simulink model "cstr_close"  (R2020b)
settings: Solver=ode15s  StartTime=0.0  StopTime=1200  RelTol=1e-8  EnableMultiTasking=on
libraries: simulink x10, pid_lib x1
settings Model: Creator=Karl  LastModifiedBy=Fuzz4
settings DataIOCC: SaveFormat=Array  ReturnWorkspaceOutputs=off  OutputOption=SpecifiedOutputTimes  OutputTimes=[0:1200]
settings OptimizationCC: LifeSpan=inf
settings DebuggingCC: UnderspecifiedInitializationDetection=Classic  MergeDetectMultiDrivingBlocksExec=none  SFUnexpectedBacktrackingDiag=warning  SFNoUnconditionalDefaultTransitionDiag=warning  SFExecutionAtInitializationDiag=none  ArithmeticOperatorsInVariantConditions=warning
settings HardwareCC: ProdBitPerPointer=32  ProdBitPerSizeT=32  ProdBitPerPtrDiffT=32  ProdLargestAtomicFloat=None  ProdIntDivRoundTo=Undefined  ProdEndianess=Unspecified  ProdWordSize=32  ProdHWDeviceType=32-bit Generic
settings ModelReferenceCC: PropagateSignalLabelsOutOfModel=off
settings SFSimCC: SimUseLocalCustomCode=off  CustomCodeUndefinedFunction=UseInterfaceOnly
settings RTWCC: RTWUseLocalCustomCode=off
settings CodeAppCC: StateflowObjectComments=on
settings GRTTargetCC: TargetLangStandard=C89/C90 (ANSI)
settings ConfigComp: CovMetricSettings=dw  CovSaveCumulativeToWorkspaceVar=on  CovSaveSingleToWorkspaceVar=on  CovExternalEMLEnable=off

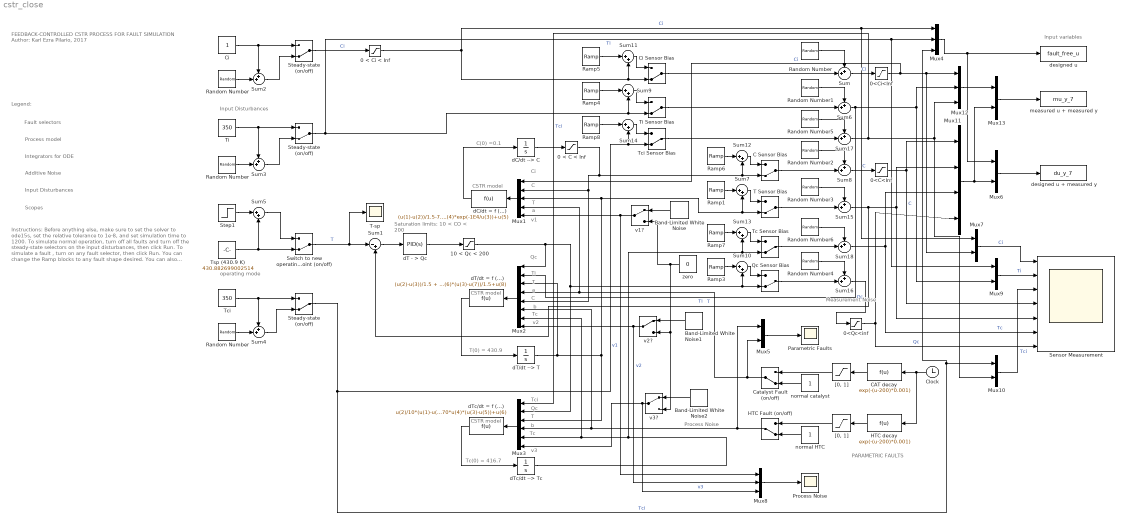
== system cstr_close ==
  note: Scopes
  note: Input Disturbances
  note: Instructions:
      |
      | Before anything else, make sure to set the solver to ode15s, set the relative tolerance to 1e-8, and set simulation time to 1200.
      |
      | To simulate normal operation, turn off all faults and turn off the steady-state selectors on the input disturbances, then click Run.
      |
      | To simulate a fault , turn on any fault selector, then click Run. You can change the Ramp blocks to any fault shape desired. You can also induce different disturbances by changing the Random Number blocks.
      |
      | Process Model:
  note: Additive Noise
  note: Integrators for ODE
  note: Process model
  note: Fault selectors
  note: Legend:
  note: FEEDBACK-CONTROLLED
      | CSTR PROCESS FOR
      | FAULT SIMULATION
      |
      | Author: Karl Ezra Pilario, 2017
  note: PARAMETRIC FAULTS
  note: v3
  note: v2
  note: v1
  note: Input variables
  note: T
  note: Tc(0) = 416.7
  note: Tc
  note: Qc
  note: Tc
  note: b
  note: Tci
  note: T
  note: Saturation limits:
      |  10 < CO < 200
  note: b
  note: CSTR model
  note: CSTR model
  note: T(0) = 430.9
  note: C(0) =0.1
  note: Measurement
      |         Noise
  note: Qc
  note: C
  note: a
  note: T
  note: Ti
  note: a
  note: C
  note: Ci
  note: CSTR model
  note: Process Noise
  note: Input Disturbances
  note: operating mode
  "   Steady-state (on/off)" : ManualSwitch  CurrentSetting=0
  "  Steady-state (on/off)" : ManualSwitch  CurrentSetting=0
  " Parametric Faults" : Scope
  " Process Noise" : Scope
  " Random Number" : RandomNumber  Seed=randi(100000)  SampleTime=60
  " [0, 1]" : Saturate  UpperLimit=1  LowerLimit=0
  0 < C < Inf : Saturate  UpperLimit=Inf  LowerLimit=0
  0 < Ci < Inf : Saturate  UpperLimit=Inf  LowerLimit=0
  0<C<Inf : Saturate  UpperLimit=Inf  LowerLimit=0
  0<Ci<Inf : Saturate  UpperLimit=Inf  LowerLimit=0
  0<Qc<inf : Saturate  UpperLimit=Inf  LowerLimit=0
  10 < Qc < 200 : Saturate  UpperLimit=200  LowerLimit=10
  Band-Limited White Noise : simulink/Sources/Band-Limited White Noise  Cov=[1e-4]  Ts=1  seed=randi(100000)
  Band-Limited White Noise1 : simulink/Sources/Band-Limited White Noise  Cov=[1e-4]  Ts=1  seed=randi(100000)
  Band-Limited White Noise2 : simulink/Sources/Band-Limited White Noise  Cov=[1e-4]  Ts=1  seed=randi(100000)
  C Sensor Bias : ManualSwitch  CurrentSetting=0
  CAT decay : Fcn  Expr=exp(-(u-200)*0.001)
  Catalyst Fault (on/off) : ManualSwitch  CurrentSetting=0
  Ci : Constant
  Ci Sensor Bias : ManualSwitch  CurrentSetting=0
  Clock : Clock
  HTC Fault (on/off) : ManualSwitch  CurrentSetting=0
  HTC decay : Fcn  Expr=exp(-(u-200)*0.001)
  Mux1 : Mux  Inputs=5
  Mux{5..7,9..10,13} (6 alike) : Mux  Inputs=2
  Mux11 : Mux
  Mux12 : Mux  Inputs=3
  Mux2 : Mux  Inputs=8
  Mux3 : Mux  Inputs=6
  Mux4 : Mux  Inputs=3
  Mux8 : Mux  Inputs=3
  Qc Sensor Bias : ManualSwitch  CurrentSetting=0
  Ramp1 : simulink/Sources/Ramp  slope=50/(1200-200)  start=200  InitialOutput=0
  Ramp3 : simulink/Sources/Ramp  slope=-100/(1200-200)  start=200  InitialOutput=0
  Ramp4 : simulink/Sources/Ramp  slope=150/(1200-200)  start=200  InitialOutput=0
  Ramp5 : simulink/Sources/Ramp  slope=2/(1200-200)  start=200  InitialOutput=0
  Ramp6 : simulink/Sources/Ramp  slope=1/(1200-200)  start=200  InitialOutput=0
  Ramp7 : simulink/Sources/Ramp  slope=50/(1200-200)  start=200  InitialOutput=0
  Ramp8 : simulink/Sources/Ramp  slope=100/(1200-200)  start=200  InitialOutput=0
  Random Number : RandomNumber  Variance=0.000001  Seed=randi(100000)  SampleTime=1
  Random Number1 : RandomNumber  Variance=0.05  Seed=randi(100000)  SampleTime=1
  Random Number2 : RandomNumber  Variance=0.000001  Seed=randi(100000)  SampleTime=1
  Random Number3 : RandomNumber  Variance=0.001  Seed=randi(100000)  SampleTime=1
  Random Number4 : RandomNumber  Variance=0.2  Seed=randi(100000)  SampleTime=1
  Random Number5 : RandomNumber  Variance=0.05  Seed=randi(100000)  SampleTime=1
  Random Number6 : RandomNumber  Variance=0.05  Seed=randi(100000)  SampleTime=1
  Random Number : RandomNumber  Variance=0.5  Seed=randi(100000)  SampleTime=60
  Random Number : RandomNumber  Variance=0.002  Seed=randi(100000)  SampleTime=60
  "Sensor Measurement " : Scope  NumInputPorts=7
  Steady-state (on/off) : ManualSwitch  CurrentSetting=0
  Step1 : Step  Time=300  After=10  SampleTime=0
  Sum{,2..4,6,8,15..18} (10 alike) : Sum  Inputs=++|
  Sum1 : Sum  Inputs=|-+
  Sum{5,7,9..14} (8 alike) : Sum  Inputs=|++
  Switch to new operating point (on/off) : ManualSwitch  CurrentSetting=0
  T Sensor Bias : ManualSwitch  CurrentSetting=0
  T-sp : Scope
  Tc Sensor Bias : ManualSwitch  CurrentSetting=0
  Tci : Constant  Value=350
  Tci Sensor Bias : ManualSwitch  CurrentSetting=0
  Ti : Constant  Value=350
  Ti Sensor Bias : ManualSwitch  CurrentSetting=0
  Tsp (430.9 K) : Constant  Value=430.882699002514
  "[0, 1]" : Saturate  UpperLimit=1  LowerLimit=0
  dC/dt --> C : Integrator  InitialCondition=0.1
  dC/dt = f (...) : Fcn  Expr=(u(1)-u(2))/1.5-7.2E10*u(2)*u(4)*exp(-1E4/u(3))+u(5)
  dT - > Qc : pid_lib/PID Controller  Controller=PID  Form=Parallel  TimeDomain=Continuous-time  UseExternalTs=off  SampleTime=-1  IntegratorMethod=Forward Euler  FilterMethod=Forward Euler  ControllerParametersSource=internal  P=1  I=5  D=0  UseFilter=on  N=100  TunerSelectOption=Transfer Function Based (PID Tuner App)  InitialConditionSource=internal  InitialConditionForIntegrator=148.550238092053  InitialConditionForFilter=0  DifferentiatorICPrevScaledInput=0  ExternalReset=none  TrackingMode=off  Kt=1  LimitOutput=on  SatLimitsSource=internal  UpperSaturationLimit=200  LowerSaturationLimit=10  LinearizeAsGain=on  AntiWindupMode=none  Kb=1  POutMin=[]  POutMax=[]  IOutMin=[]  IOutMax=[]  DOutMin=[]  DOutMax=[]  NOutMin=[]  NOutMax=[]  SumOutMin=[]  SumOutMax=[]  SaturationOutMin=[]  SaturationOutMax=[]  PParamMin=[]  PParamMax=[]  IParamMin=[]  IParamMax=[]  DParamMin=[]  DParamMax=[]  NParamMin=[]  NParamMax=[]  KbParamMin=[]  KbParamMax=[]  KtParamMin=[]  KtParamMax=[]  KbOutMin=[]  KbOutMax=[]  KtOutMin=[]  KtOutMax=[]  IntegratorOutMin=[]  IntegratorOutMax=[]  FilterOutMin=[]  FilterOutMax=[]  SumI1OutMin=[]  SumI1OutMax=[]  SumI2OutMin=[]  SumI2OutMax=[]  SumI3OutMin=[]  SumI3OutMax=[]  SumI4OutMin=[]  SumI4OutMax=[]  SumDOutMin=[]  SumDOutMax=[]  DifferentiatorOutMin=[]  DifferentiatorOutMax=[]  FilterDiffOutCoefMin=[]  FilterDiffOutCoefMax=[]  ReciprocalOutMin=[]  ReciprocalOutMax=[]  SumDenOutMin=[]  SumDenOutMax=[]  SumNumOutMin=[]  SumNumOutMax=[]  DivideOutMin=[]  DivideOutMax=[]  UdiffTsProdOutMin=[]  UdiffTsProdOutMax=[]  NTsProdOutMin=[]  NTsProdOutMax=[]  UintegralTsProdOutMin=[]  UintegralTsProdOutMax=[]  UngainTsProdOutMin=[]  UngainTsProdOutMax=[]  IntegratorContinuousStateAttributes=''  IntegratorStateMustResolveToSignalObject=off  IntegratorRTWStateStorageClass=Auto  FilterContinuousStateAttributes=''  FilterStateMustResolveToSignalObject=off  FilterRTWStateStorageClass=Auto  ParallelPVariant=InternalParameters  IdealPVariant=Disabled  IVariant=InternalParameters  DVariant=InternalParameters  IntegratorVariant=Continuous  SatVariant=Enabled  AWVariant=Passthrough  PCopyVariant=Disabled  TRVariant=Disabled  FdbkBlocksVariant=Forward  IdealPFdbkVariant=Disabled  SatFdbkVariant=Disabled  DerivativeFilterVariant=ContFilter  NVariant=InternalParameters  NCopyVariant=Disabled  FilterICVariant=InternalICsFilter  IntegratorICVariant=InternalICs  ExternalResetVariant=Disabled  TRSumVariant=Passthrough  SumFdbkVariant=Disabled  SumVariant=Sum_PID  TsampFilterVariant=InternalTs  TsampNgainVariant=Passthrough  TsampIntegralVariant=Passthrough  ExternalSaturationOutDataTypeStr=Inherit: Same as second input
  dT/dt --> T : Integrator  InitialCondition=430.882699002514
  dT/dt = f (...) : Fcn  Expr=(u(2)-u(3))/1.5 + u(4)*7.2E10*exp(-1E4/u(3))*u(5)*2E2 - 7*u(6)*(u(3)-u(7))/1.5+u(8)
  dTc/dt --> Tc : Integrator  InitialCondition=416.723084574301
  dTc/dt = f (...) : Fcn  Expr=u(2)/10*(u(1)-u(5)) + 70*u(4)*(u(3)-u(5))+u(6)
  designed u : ToWorkspace  VariableName=fault_free_u  SampleTime=1
  designed u + measured y : ToWorkspace  VariableName=du_y_7  SampleTime=-1
  measured u + measured y : ToWorkspace  VariableName=mu_y_7  SampleTime=-1
  normal catalyst : Constant
  normal HTC : Constant
  v1? : ManualSwitch
  v2? : ManualSwitch
  v3? : ManualSwitch
  zero : Constant  Value=0
  wires:
  dT/dt = f (...)/1 -> dT/dt --> T/1
  Mux1/1 -> dC/dt = f (...)/1
  Catalyst Fault (on/off)/1 -> Mux5/2, Mux1/4, Mux2/4
  Mux2/1 -> dT/dt = f (...)/1
  dT/dt --> T/1 -> Mux2/3, Mux1/3, Sum7/2, T Sensor Bias/2, Mux3/3
  Sum1/1 -> dT - > Qc/1
  CAT decay/1 -> "[0, 1]"/1
  Ci/1 -> Steady-state (on/off)/1, Sum2/1
  Ti/1 -> "  Steady-state (on/off)"/1, Sum3/1
  normal catalyst/1 -> Catalyst Fault (on/off)/2
  HTC Fault (on/off)/1 -> Mux5/1, Mux2/6, Mux3/4
  Sum2/1 -> Steady-state (on/off)/2
  Sum3/1 -> "  Steady-state (on/off)"/2
  Switch to new operating point (on/off)/1 -> T-sp/1, Sum1/1  "T"
  Tsp (430.9 K)/1 -> Sum5/2, Switch to new operating point (on/off)/2
  Clock/1 -> HTC decay/1, CAT decay/1
  HTC decay/1 -> " [0, 1]"/1
  Tci/1 -> "   Steady-state (on/off)"/1, Sum4/1
  Sum4/1 -> "   Steady-state (on/off)"/2
  Mux3/1 -> dTc/dt = f (...)/1
  dTc/dt = f (...)/1 -> dTc/dt --> Tc/1
  dTc/dt --> Tc/1 -> Mux2/7, Mux3/5, Sum13/2, Tc Sensor Bias/2
  Sum18/1 -> Mux11/3, "Sensor Measurement "/6  "Tc"
  Sum17/1 -> Mux10/2, Mux12/3, Mux3/1  "Tci"
  0<Qc<inf/1 -> Mux11/4, "Sensor Measurement "/7  "Qc"
  Mux11/1 -> Mux6/2, Mux13/2
  Mux5/1 -> " Parametric Faults"/1
  0 < Ci < Inf/1 -> Sum11/2, Ci Sensor Bias/2, Mux7/1, Mux4/1  "Ci"
  0<Ci<Inf/1 -> Mux7/2, Mux12/1, Mux1/1  "Ci"
  0 < C < Inf/1 -> Mux2/5, Mux1/2, Sum12/2, C Sensor Bias/2
  Sum9/1 -> Ti Sensor Bias/1
  Ramp4/1 -> Sum9/1
  dC/dt = f (...)/1 -> dC/dt --> C/1
  Ramp3/1 -> Sum10/1
  Sum10/1 -> Qc Sensor Bias/1
  Ci Sensor Bias/1 -> Sum/2
  Sum11/1 -> Ci Sensor Bias/1
  Ramp1/1 -> Sum7/1
  Sum7/1 -> T Sensor Bias/1
  C Sensor Bias/1 -> Sum8/2
  Sum12/1 -> C Sensor Bias/1
  Ramp6/1 -> Sum12/1
  Tc Sensor Bias/1 -> Sum18/2
  Sum13/1 -> Tc Sensor Bias/1
  Ramp7/1 -> Sum13/1
  Sum14/1 -> Tci Sensor Bias/1
  Ramp8/1 -> Sum14/1
  Sum5/1 -> Switch to new operating point (on/off)/1
  Step1/1 -> Sum5/1
  Mux8/1 -> " Process Noise"/1
  Band-Limited White Noise/1 -> v1?/1
  v1?/1 -> Mux8/1, Mux1/5  "v1"
  Band-Limited White Noise1/1 -> v2?/1
  v2?/1 -> Mux8/2, Mux2/8  "v2"
  Band-Limited White Noise2/1 -> v3?/1
  v3?/1 -> Mux8/3, Mux3/6  "v3"
  zero/1 -> v1?/2, v3?/2, v2?/2
  normal HTC/1 -> HTC Fault (on/off)/2
  Ramp5/1 -> Sum11/1
  10 < Qc < 200/1 -> Mux2/1, Sum10/2, Qc Sensor Bias/2, Mux3/2
  Random Number/1 -> Sum2/2
  Random Number/1 -> Sum3/2
  " Random Number"/1 -> Sum4/2
  " [0, 1]"/1 -> HTC Fault (on/off)/1
  "[0, 1]"/1 -> Catalyst Fault (on/off)/1
  0<C<Inf/1 -> Mux11/1, "Sensor Measurement "/4  "C"
  Sum15/1 -> Mux11/2, "Sensor Measurement "/5, Sum1/2  "T"
  Random Number/1 -> Sum/1
  Random Number1/1 -> Sum6/1
  Ti Sensor Bias/1 -> Sum6/2
  Sum6/1 -> Mux9/2, Mux12/2, Mux2/2  "Ti"
  Random Number2/1 -> Sum8/1
  T Sensor Bias/1 -> Sum15/2
  Random Number3/1 -> Sum15/1
  Qc Sensor Bias/1 -> Sum16/2
  Random Number4/1 -> Sum16/1
  Tci Sensor Bias/1 -> Sum17/2
  Random Number5/1 -> Sum17/1
  Random Number6/1 -> Sum18/1
  "  Steady-state (on/off)"/1 -> Sum9/2, Ti Sensor Bias/2, Mux9/1, Mux4/2  "Ti"
  "   Steady-state (on/off)"/1 -> Tci Sensor Bias/2, Sum14/2, Mux4/3, Mux10/1  "Tci"
  Mux7/1 -> "Sensor Measurement "/1  "Ci"
  Mux9/1 -> "Sensor Measurement "/2  "Ti"
  Mux10/1 -> "Sensor Measurement "/3  "Tci"
  Mux4/1 -> Mux6/1, designed u/1
  Mux12/1 -> Mux13/1
  Mux13/1 -> measured u + measured y/1
  dT - > Qc/1 -> 10 < Qc < 200/1
  Sum16/1 -> 0<Qc<inf/1  "Qc"
  Steady-state (on/off)/1 -> 0 < Ci < Inf/1  "Ci"
  dC/dt --> C/1 -> 0 < C < Inf/1
  Sum/1 -> 0<Ci<Inf/1  "Ci"
  Sum8/1 -> 0<C<Inf/1  "C"
  Mux6/1 -> designed u + measured y/1
